simulink model "gs_integracion"  (Simulink 7.5)
settings: Solver=ode45  StartTime=0.0  StopTime=50  RelTol=1e-3
settings Model: Creator=Fer  LastModifiedBy=Fer

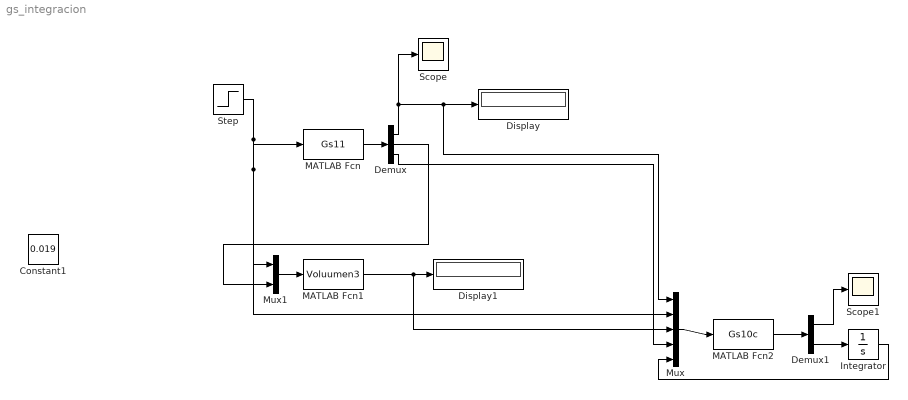
== system gs_integracion ==
  Constant1 : Constant  Value=0.019  OutDataType=fixdt(1, 16)  OutScaling=2^0
  Demux : Demux  Outputs=3
  Demux1 : Demux  Outputs=2
  Display : Display
  Display1 : Display
  Integrator : Integrator  InitialCondition=1.6
  MATLAB Fcn : MATLABFcn  MATLABFcn=Gs11
  MATLAB Fcn1 : MATLABFcn  MATLABFcn=Voluumen3
  MATLAB Fcn2 : MATLABFcn  MATLABFcn=Gs10c
  Mux : Mux  Inputs=5
  Mux1 : Mux  Inputs=2
  Scope : Scope
  Scope1 : Scope
  Step : Step  Time=30  Before=0.019  After=0.9  SampleTime=0
  wires:
  Step/1 -> MATLAB Fcn/1, Mux1/1, Mux/2
  Mux1/1 -> MATLAB Fcn1/1
  MATLAB Fcn/1 -> Demux/1
  Demux/1 -> Scope/1, Display/1, Mux/1
  Demux/2 -> Mux1/2
  MATLAB Fcn1/1 -> Display1/1, Mux/3
  Mux/1 -> MATLAB Fcn2/1
  MATLAB Fcn2/1 -> Demux1/1
  Demux/3 -> Mux/4
  Demux1/1 -> Scope1/1
  Demux1/2 -> Integrator/1
  Integrator/1 -> Mux/5
